simulink model "New_mavsim_chap12"  (R2019b)
settings: Solver=ode45  StartTime=0.0  StopTime=70  RelTol=1e-3  EnableMultiTasking=on
InitFcn:
  | param_chap1
undefined symbols (not defined in the file or in its folder): drawEnvironment, P, path_follow1, path_follow2, path_manager1, path_manager2, path_planner1, path_planner2
settings Model: Creator=beard  LastModifiedBy=Work
settings DataIOCC: LimitDataPoints=on  SaveFormat=Array  SignalLoggingSaveFormat=ModelDataLogs  ReturnWorkspaceOutputs=off
settings OptimizationCC: ExpressionDepthLimit=2147483647  InitFltsAndDblsToZero=on  LifeSpan=inf
settings DebuggingCC: UnderspecifiedInitializationDetection=Classic  MergeDetectMultiDrivingBlocksExec=none  SolverPrmCheckMsg=warning  FcnCallInpInsideContextMsg=warning  AllowSymbolicDim=off  StateNameClashWarn=warning  SFUnexpectedBacktrackingDiag=warning  SFNoUnconditionalDefaultTransitionDiag=warning  SFExecutionAtInitializationDiag=none  ArithmeticOperatorsInVariantConditions=warning
settings HardwareCC: ProdBitPerPointer=32  ProdBitPerSizeT=32  ProdBitPerPtrDiffT=32  ProdLargestAtomicFloat=None  ProdIntDivRoundTo=Undefined  ProdEndianess=Unspecified  ProdWordSize=32  ProdHWDeviceType=32-bit Generic
settings ModelReferenceCC: PropagateSignalLabelsOutOfModel=off
settings SFSimCC: SimUseLocalCustomCode=off  SimParseCustomCode=off  CustomCodeUndefinedFunction=UseInterfaceOnly
settings RTWCC: RTWUseLocalCustomCode=off
settings CodeAppCC: StateflowObjectComments=on
settings GRTTargetCC: TargetLangStandard=C89/C90 (ANSI)  GeneratePreprocessorConditionals=Disable all  CombineOutputUpdateFcns=off  GRTInterface=on
settings ConfigComp: CovMetricSettings=dw  CovHtmlReporting=on  CovSaveCumulativeToWorkspaceVar=on  CovSaveSingleToWorkspaceVar=on  CovExternalEMLEnable=off  CovSFcnEnable=off

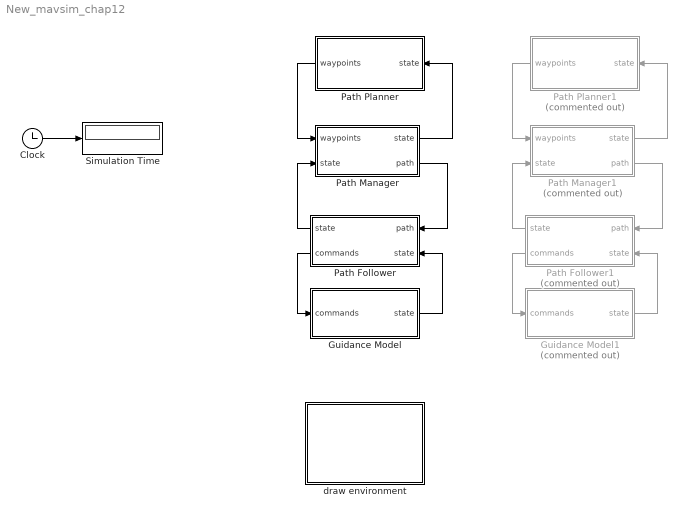
== system New_mavsim_chap12 ==
  Clock : Clock
  Guidance Model : Subsystem
  Guidance Model1 : Subsystem  Commented=on
  Path Follower : Subsystem
  Path Follower1 : Subsystem  Commented=on
  Path Manager : Subsystem
  Path Manager1 : Subsystem  Commented=on
  Path Planner : Subsystem
  Path Planner1 : Subsystem  Commented=on
  Simulation Time : Display
  draw environment : Subsystem
      mask Display: image(imread('predator.jpg'))
  wires:
  Clock/1 -> Simulation Time/1
  Path Manager/2(path) -> Path Follower/1(path)
  Path Follower/2(commands) -> Guidance Model/1(commands)
  Guidance Model/1(state) -> Path Follower/2(state)
  Path Follower/1("state ") -> Path Manager/2(state)
  Path Planner/1(waypoints) -> Path Manager/1(waypoints)
  Path Manager/1("state ") -> Path Planner/1(state)
  Path Manager1/2(path) -> Path Follower1/1(path)
  Path Follower1/2(commands) -> Guidance Model1/1(commands)
  Path Planner1/1(waypoints) -> Path Manager1/1(waypoints)
  Path Manager1/1("state ") -> Path Planner1/1(state)
  Path Follower1/1("state ") -> Path Manager1/2(state)
  Guidance Model1/1(state) -> Path Follower1/2(state)

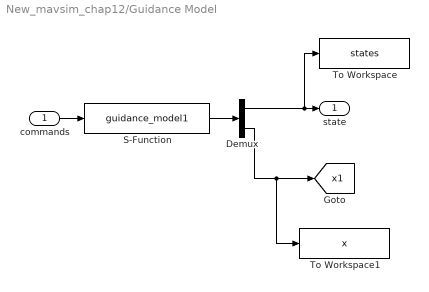
== system New_mavsim_chap12/Guidance Model ==
  commands : Inport
  Demux : Demux  Outputs=[16;12]
  S-Function : S-Function  FunctionName=guidance_model1  Parameters=P  SFunctionDeploymentMode=off  EnableBusSupport=off
  To Workspace : ToWorkspace  VariableName=states  SaveFormat=Timeseries  SampleTime=-1
  To Workspace1 : ToWorkspace  VariableName=x  SaveFormat=Timeseries  SampleTime=-1
  state : Outport
  tag scope: x1=global
  wires:
  commands/1 -> S-Function/1
  S-Function/1 -> Demux/1
  Demux/1 -> To Workspace/1, state/1
  Demux/2 -> To Workspace1/1, [x1]

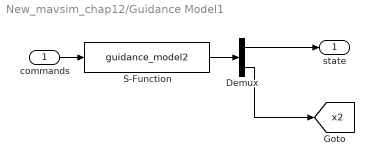
== system New_mavsim_chap12/Guidance Model1 ==
  commands : Inport
  Demux : Demux  Outputs=[16;12]
  S-Function : S-Function  FunctionName=guidance_model2  Parameters=P  SFunctionDeploymentMode=off  EnableBusSupport=off
  state : Outport
  tag scope: x2=global
  wires:
  commands/1 -> S-Function/1
  S-Function/1 -> Demux/1
  Demux/1 -> state/1
  Demux/2 -> [x2]

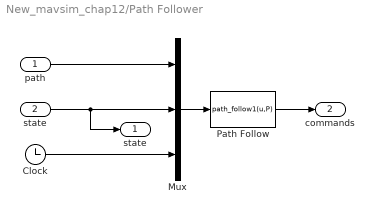
== system New_mavsim_chap12/Path Follower ==
  path : Inport
  state : Inport  Port=2
  Clock : Clock
  Mux : Mux  Inputs=3
  Path Follow : MATLABFcn  MATLABFcn=path_follow1(u,P)  OutputDimensions=4  SampleTime=P.Ts
  "state " : Outport
  commands : Outport  Port=2
  wires:
  Path Follow/1 -> commands/1
  Mux/1 -> Path Follow/1
  path/1 -> Mux/1
  Clock/1 -> Mux/3
  state/1 -> Mux/2, "state "/1

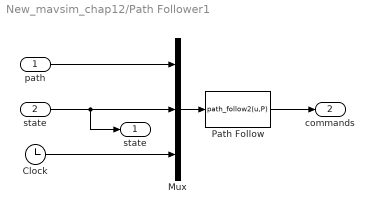
== system New_mavsim_chap12/Path Follower1 ==
  path : Inport
  state : Inport  Port=2
  Clock : Clock
  Mux : Mux  Inputs=3
  Path Follow : MATLABFcn  MATLABFcn=path_follow2(u,P)  OutputDimensions=4  SampleTime=P.Ts
  "state " : Outport
  commands : Outport  Port=2
  wires:
  Path Follow/1 -> commands/1
  Mux/1 -> Path Follow/1
  path/1 -> Mux/1
  Clock/1 -> Mux/3
  state/1 -> Mux/2, "state "/1

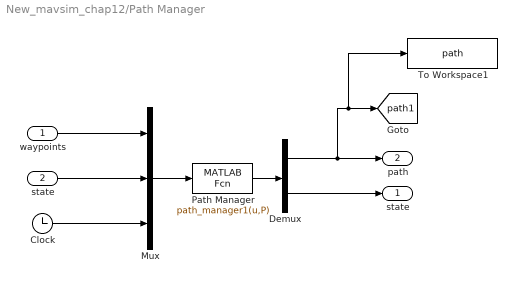
== system New_mavsim_chap12/Path Manager ==
  waypoints : Inport
  state : Inport  Port=2
  Clock : Clock
  Demux : Demux  Outputs=[13;17]
  Mux : Mux  Inputs=3
  Path Manager : MATLABFcn  MATLABFcn=path_manager1(u,P)  OutputDimensions=30  SampleTime=P.Ts
  To Workspace1 : ToWorkspace  VariableName=path  SaveFormat=Timeseries  SampleTime=-1
  "state " : Outport
  path : Outport  Port=2
  tag scope: path1=global
  wires:
  Demux/2 -> "state "/1
  Demux/1 -> To Workspace1/1, [path1], path/1
  Path Manager/1 -> Demux/1
  waypoints/1 -> Mux/1
  state/1 -> Mux/2
  Clock/1 -> Mux/3
  Mux/1 -> Path Manager/1

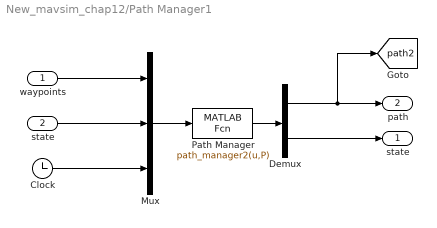
== system New_mavsim_chap12/Path Manager1 ==
  waypoints : Inport
  state : Inport  Port=2
  Clock : Clock
  Demux : Demux  Outputs=[13;17]
  Mux : Mux  Inputs=3
  Path Manager : MATLABFcn  MATLABFcn=path_manager2(u,P)  OutputDimensions=30  SampleTime=P.Ts
  "state " : Outport
  path : Outport  Port=2
  tag scope: path2=global
  wires:
  Demux/2 -> "state "/1
  Demux/1 -> [path2], path/1
  Path Manager/1 -> Demux/1
  waypoints/1 -> Mux/1
  state/1 -> Mux/2
  Clock/1 -> Mux/3
  Mux/1 -> Path Manager/1

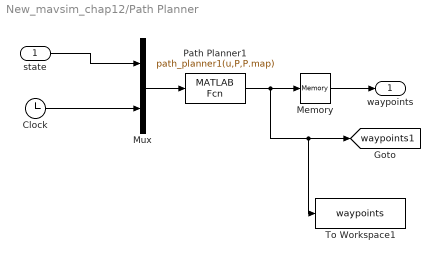
== system New_mavsim_chap12/Path Planner ==
  state : Inport
  Clock : Clock
  Memory : Memory
  Mux : Mux  Inputs=2
  Path Planner1 : MATLABFcn  MATLABFcn=path_planner1(u,P,P.map)  OutputDimensions=1+5*P.size_waypoint_array  SampleTime=100*P.Ts
  To Workspace1 : ToWorkspace  VariableName=waypoints  SaveFormat=Timeseries  SampleTime=-1
  waypoints : Outport
  tag scope: waypoints1=global
  wires:
  Mux/1 -> Path Planner1/1
  Clock/1 -> Mux/2
  state/1 -> Mux/1
  Path Planner1/1 -> Memory/1, To Workspace1/1, [waypoints1]
  Memory/1 -> waypoints/1

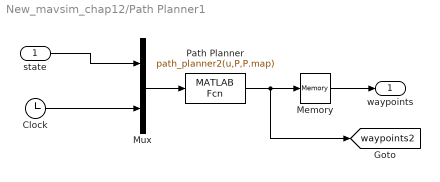
== system New_mavsim_chap12/Path Planner1 ==
  state : Inport
  Clock : Clock
  Memory : Memory
  Mux : Mux  Inputs=2
  Path Planner : MATLABFcn  MATLABFcn=path_planner2(u,P,P.map)  OutputDimensions=1+5*P.size_waypoint_array  SampleTime=100*P.Ts
  waypoints : Outport
  tag scope: waypoints2=global
  wires:
  Mux/1 -> Path Planner/1
  Clock/1 -> Mux/2
  state/1 -> Mux/1
  Path Planner/1 -> Memory/1, [waypoints2]
  Memory/1 -> waypoints/1

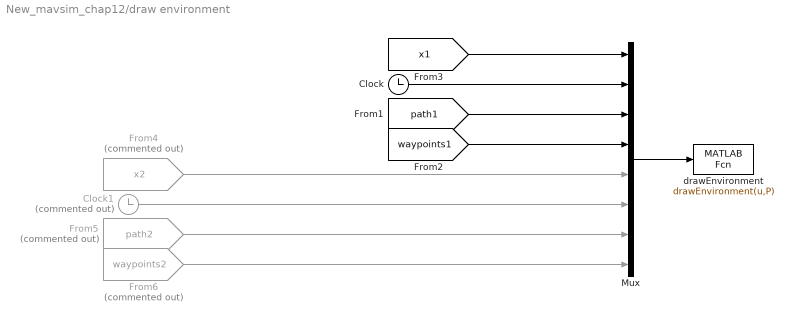
== system New_mavsim_chap12/draw environment ==
  Clock : Clock
  Clock1 : Clock  Commented=on
  From4 : From  Commented=on  GotoTag=x2  TagVisibility=global
      settings: CloseFcn=tagdialog Close
  From5 : From  Commented=on  GotoTag=path2  TagVisibility=global
      settings: CloseFcn=tagdialog Close
  From6 : From  Commented=on  GotoTag=waypoints2  TagVisibility=global
      settings: CloseFcn=tagdialog Close
  Mux : Mux  Inputs=8
  drawEnvironment : MATLABFcn  MATLABFcn=drawEnvironment(u,P)  OutputDimensions=0  SampleTime=0.1
  wires:
  Clock/1 -> Mux/2
  [x1] -> Mux/1
  Mux/1 -> drawEnvironment/1
  [path1] -> Mux/3
  [waypoints1] -> Mux/4
  From5/1 -> Mux/7
  From6/1 -> Mux/8
  Clock1/1 -> Mux/6
  From4/1 -> Mux/5
